simulink model "Observable_System"  (R2016a)
settings: Solver=ode45  StartTime=0.0  StopTime=10.0  RelTol=1e-3
values from neighbouring files (symbols this model uses):
  A = [0,1,0,0;20.9,0,0,0;0,0,0,1;-0.8,0,0,0]    [SSAE_script.m]
  B = [0;-1;0;0.5]    [SSAE_script.m]
  C = [1,0,0,0;0,0,1,0]    [SSAE_script.m]
  K_Obs = place(A',C',poles)'    [SSAE_script.m]
settings Model: Creator=el12074  LastModifiedBy=dimst
settings DataIOCC: LimitDataPoints=on  SaveFormat=Array
settings DebuggingCC: SolverPrmCheckMsg=warning
settings HardwareCC: ProdBitPerPointer=32  ProdLargestAtomicFloat=None  ProdIntDivRoundTo=Undefined  ProdEndianess=Unspecified  ProdWordSize=32  ProdHWDeviceType=32-bit Generic
settings ModelReferenceCC: PropagateSignalLabelsOutOfModel=off
settings ConfigComp: CovModelRefEnable=Off  CovSFcnEnable=off

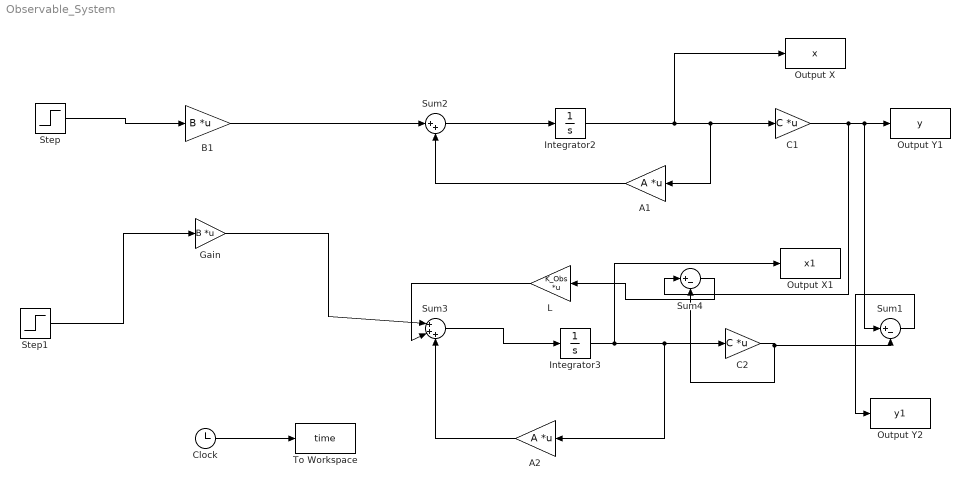
== system Observable_System ==
  A1 : Gain  Gain=A  Multiplication=Matrix(K*u)
  A2 : Gain  Gain=A  Multiplication=Matrix(K*u)
  B1 : Gain  Gain=B  Multiplication=Matrix(K*u)
  C1 : Gain  Gain=C  Multiplication=Matrix(K*u)
  C2 : Gain  Gain=C  Multiplication=Matrix(K*u)
  Clock : Clock
  Gain : Gain  Gain=B  Multiplication=Matrix(K*u)
  Integrator2 : Integrator  InitialCondition=[-0.2;-0.06;0.01;0.3]
  Integrator3 : Integrator  InitialCondition=[0;0;0;0]
  L : Gain  Gain=K_Obs  Multiplication=Matrix(K*u)
  Output X : ToWorkspace  VariableName=x  SampleTime=-1
      settings: Save2DSignal=2-D array (concatenate along first dimension)
  Output X1 : ToWorkspace  VariableName=x1  SampleTime=-1
      settings: Save2DSignal=2-D array (concatenate along first dimension)
  Output Y1 : ToWorkspace  VariableName=y  SampleTime=-1
      settings: Save2DSignal=2-D array (concatenate along first dimension)
  Output Y2 : ToWorkspace  VariableName=y1  SampleTime=-1
      settings: Save2DSignal=2-D array (concatenate along first dimension)
  Step : Step  SampleTime=0
  Step1 : Step  SampleTime=0
  Sum1 : Sum  Inputs=|+-
  Sum2 : Sum  Inputs=|++
  Sum3 : Sum  Inputs=|+++
  Sum4 : Sum  Inputs=|+-
  To Workspace : ToWorkspace  VariableName=time  SampleTime=-1
      settings: Save2DSignal=2-D array (concatenate along first dimension)
  wires:
  Clock/1 -> To Workspace/1
  B1/1 -> Sum2/1
  A1/1 -> Sum2/2
  Sum2/1 -> Integrator2/1
  Integrator2/1 -> Output X/1, C1/1, A1/1
  C1/1 -> Sum4/1, Sum1/1, Output Y1/1
  Gain/1 -> Sum3/1
  L/1 -> Sum3/2
  A2/1 -> Sum3/3
  Sum3/1 -> Integrator3/1
  Integrator3/1 -> Output X1/1, A2/1, C2/1
  Sum4/1 -> L/1
  C2/1 -> Sum1/2, Sum4/2
  Step/1 -> B1/1
  Step1/1 -> Gain/1
  Sum1/1 -> Output Y2/1
